simulink model "PersonFollower_TestModule"  (R2023b)
settings: Solver=FixedStepAuto  StartTime=0.0  StopTime=inf  FixedStep=1  RelTol=1e-3
model workspace (MAT data in the model file):
  SL_ROS_VariableLengthArrays_MaxSizes.CommonInfo.ArrayTruncateAction = 'EmitWarning'
  SL_ROS_VariableLengthArrays_MaxSizes.MsgTypeMap = containers.Map
  SL_ROS_VariableLengthArrays_MaxSizes.MsgTypeMap.serialization.keys = {'sensor_msgs/CompressedImage', 'sensor_msgs/LaserScan'}
  SL_ROS_VariableLengthArrays_MaxSizes.MsgTypeMap.serialization.values{1}(1).PropertyName = 'data'
  SL_ROS_VariableLengthArrays_MaxSizes.MsgTypeMap.serialization.values{1}(1).DataType = 'uint8'
  SL_ROS_VariableLengthArrays_MaxSizes.MsgTypeMap.serialization.values{1}(1).MaxLength = 300000
  SL_ROS_VariableLengthArrays_MaxSizes.MsgTypeMap.serialization.values{1}(2).PropertyName = 'format'
  SL_ROS_VariableLengthArrays_MaxSizes.MsgTypeMap.serialization.values{1}(2).DataType = 'uint8'
  SL_ROS_VariableLengthArrays_MaxSizes.MsgTypeMap.serialization.values{1}(2).MaxLength = 128
  SL_ROS_VariableLengthArrays_MaxSizes.MsgTypeMap.serialization.values{2}(1).PropertyName = 'intensities'
  SL_ROS_VariableLengthArrays_MaxSizes.MsgTypeMap.serialization.values{2}(1).DataType = 'single'
  SL_ROS_VariableLengthArrays_MaxSizes.MsgTypeMap.serialization.values{2}(1).MaxLength = 2000
  SL_ROS_VariableLengthArrays_MaxSizes.MsgTypeMap.serialization.values{2}(2).PropertyName = 'ranges'
  SL_ROS_VariableLengthArrays_MaxSizes.MsgTypeMap.serialization.values{2}(2).DataType = 'single'
  SL_ROS_VariableLengthArrays_MaxSizes.MsgTypeMap.serialization.values{2}(2).MaxLength = 2000
  SL_ROS_VariableLengthArrays_MaxSizes.MsgTypeMap.serialization.uniformity = 0
  SL_ROS_VariableLengthArrays_MaxSizes.MsgTypeMap.serialization.keyType = 'char'
  SL_ROS_VariableLengthArrays_MaxSizes.MsgTypeMap.serialization.valueType = 'any'
undefined symbols (not defined in the file or in its folder): angular, linear
libraries: ros2lib x6, simulink_extras x1, simulink x1
settings Model: Creator=bowen  LastModifiedBy=bowen
settings OptimizationCC: EnhancedBackFolding=on  PassReuseOutputArgsAs=Individual arguments  ZeroExternalMemoryAtStartup=off  ZeroInternalMemoryAtStartup=off  MaxStackSize=64  OptimizeBlockOrder=speed  DifferentSizesBufferReuse=on  OptimizationCustomize=off  EfficientTunableParamExpr=on
settings DebuggingCC: ParameterTunabilityLossMsg=error
settings SFSimCC: MATLABDynamicMemAlloc=off
settings RTWCC: Description=Embedded Coder  SystemTargetFile=ert.tlc  HardwareBoard=Robot Operating System 2 (ROS 2)  TLCOptions="-aInlineSetEventsForThisBaseRateFcn=TLC_FALSE -aSuppressMultiTaskScheduler=TLC_FALSE  -aRateBasedStepFcn=0"  TemplateMakefile=ert_default_tmf  Toolchain=Colcon Tools  TargetLang=C++
settings CodeAppCC: ForceParamTrailComments=on  IgnoreCustomStorageClasses=off  OperatorAnnotations=on  SimulinkDataObjDesc=on  SFDataObjDesc=on  InsertBlockDesc=on
settings ERTTargetCC: CodeInterfacePackaging=C++ class  RootIOFormat=Structure reference

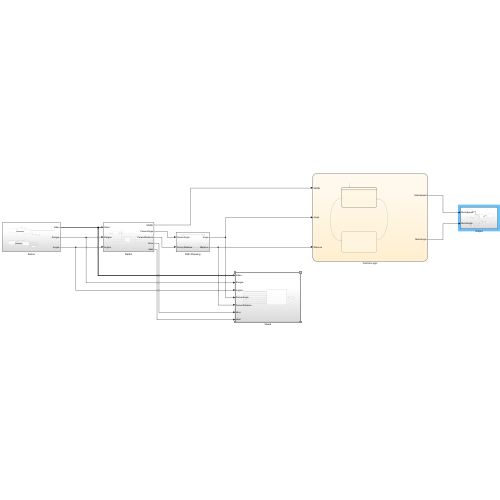
[thumbnail: Simulink's stored preview of the top-level diagram]
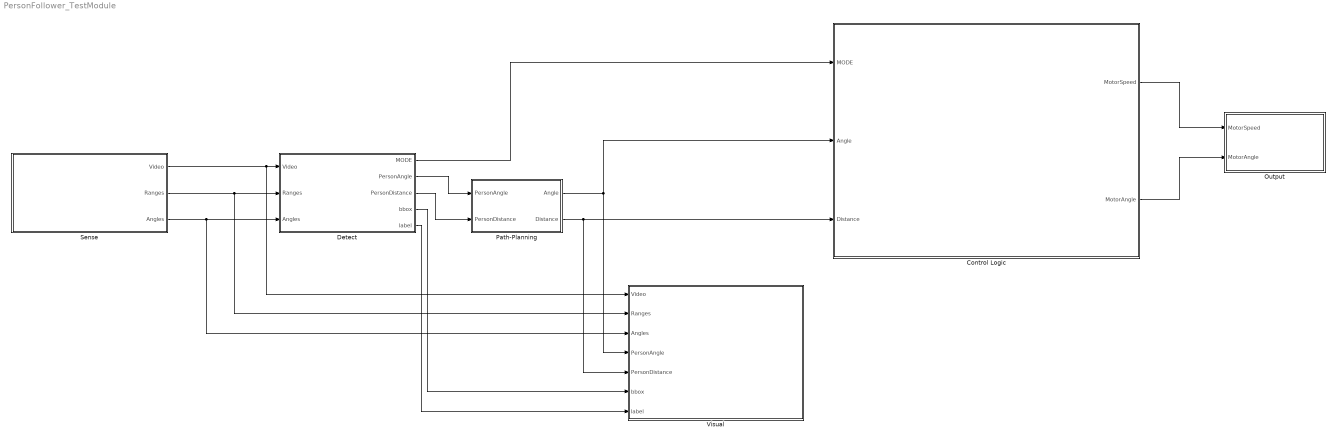
== system PersonFollower_TestModule ==
  Control Logic : Stateflow chart  TreatAsAtomicUnit=on
  Detect : Subsystem
  Output : Subsystem
  Path-Planning : Subsystem
  Sense : Subsystem
  Visual : Subsystem
  wires:
  Sense/1(Video) -> Visual/1(Video), Detect/1(Video)
  Sense/2(Ranges) -> Visual/2(Ranges), Detect/2(Ranges)
  Sense/3(Angles) -> Visual/3(Angles), Detect/3(Angles)
  Detect/1(MODE) -> Control Logic/1(MODE)
  Control Logic/1(MotorSpeed) -> Output/1(MotorSpeed)
  Control Logic/2(MotorAngle) -> Output/2(MotorAngle)
  Detect/2(PersonAngle) -> Path-Planning/1("PersonAngle ")
  Detect/3(PersonDistance) -> Path-Planning/2(PersonDistance)
  Path-Planning/1(Angle) -> Control Logic/2(Angle), Visual/4(PersonAngle)
  Path-Planning/2(Distance) -> Visual/5(PersonDistance), Control Logic/3(Distance)
  Detect/4(bbox) -> Visual/6(bbox)
  Detect/5(label) -> Visual/7(label)

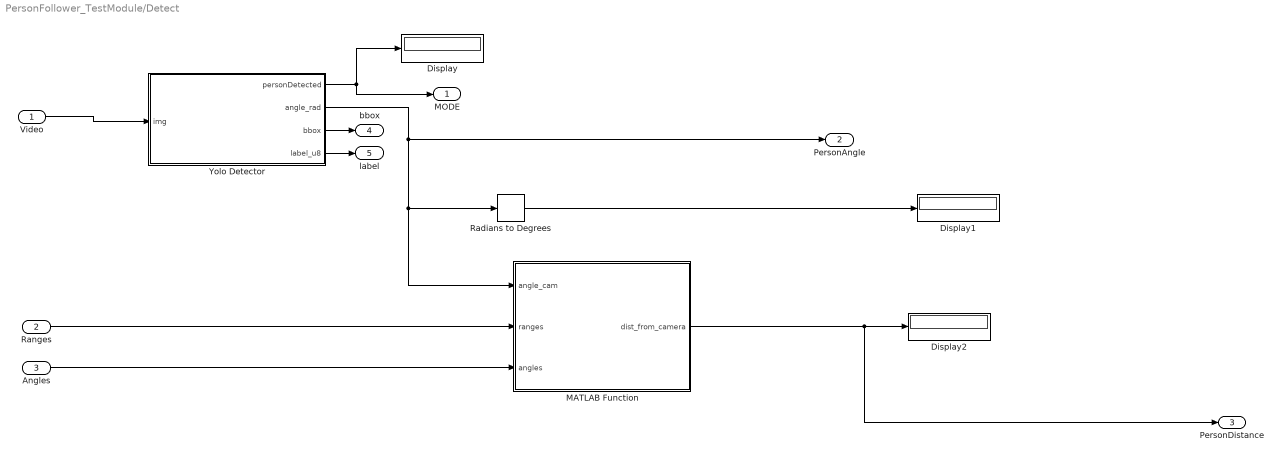
== system PersonFollower_TestModule/Detect ==
  Video : Inport
  Ranges : Inport  Port=2
  Angles : Inport  Port=3
  Display : Display
  Display1 : Display
  Display2 : Display
  MATLAB Function : MATLAB Function  TreatAsAtomicUnit=on
  Radians to Degrees : simulink_extras/Transformations/Radians to Degrees
  Yolo Detector : MATLAB Function  TreatAsAtomicUnit=on
  MODE : Outport
  PersonAngle : Outport  Port=2
  PersonDistance : Outport  Port=3
  bbox : Outport  Port=4
  label : Outport  Port=5
  wires:
  Video/1 -> Yolo Detector/1(img)
  Yolo Detector/1(personDetected) -> MODE/1, Display/1
  Yolo Detector/2(angle_rad) -> MATLAB Function/1(angle_cam), Radians to Degrees/1, PersonAngle/1
  Ranges/1 -> MATLAB Function/2(ranges)
  Angles/1 -> MATLAB Function/3(angles)
  Radians to Degrees/1 -> Display1/1
  MATLAB Function/1(dist_from_camera) -> PersonDistance/1, Display2/1
  Yolo Detector/3(bbox) -> bbox/1
  Yolo Detector/4(label_u8) -> label/1

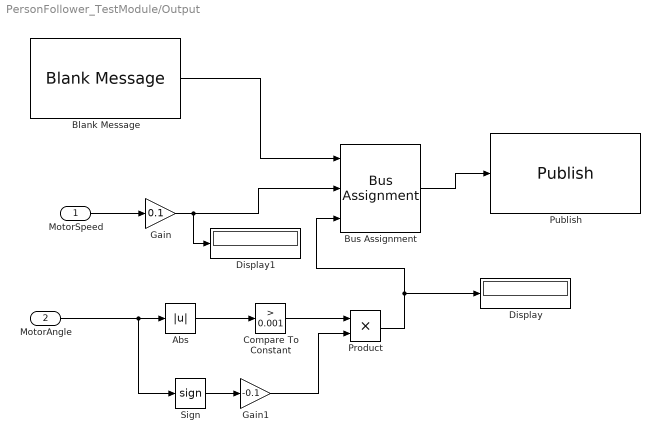
== system PersonFollower_TestModule/Output ==
  MotorSpeed : Inport
  MotorAngle : Inport  Port=2
  Abs : Abs  SaturateOnIntegerOverflow=off
  Blank Message : ros2lib/Blank Message  messageClass=Message  entityType=geometry_msgs/Twist  messageType=geometry_msgs/Twist  SampleTime=1
  Bus Assignment : BusAssignment  AssignedSignals=linear.x,angular.z
  Compare To Constant : simulink/Logic and Bit Operations/Compare To Constant  relop=>  const=0.001  OutDataTypeStr=boolean
  Display : Display
  Display1 : Display
  Gain : Gain  Gain=0.1
  Gain1 : Gain  Gain=-0.1
  Product : Product
  Publish : ros2lib/Publish  topicSource=Select from ROS network  topic=/controller/cmd_vel  messageType=geometry_msgs/Twist  QOSHistory=Keep last  QOSDepth=1  QOSReliability=Reliable  QOSDurability=Volatile
  Sign : Signum
  wires:
  Blank Message/1 -> Bus Assignment/1
  Bus Assignment/1 -> Publish/1
  Gain/1 -> Bus Assignment/2, Display1/1
  MotorSpeed/1 -> Gain/1
  MotorAngle/1 -> Sign/1, Abs/1
  Abs/1 -> Compare To Constant/1
  Sign/1 -> Gain1/1
  Compare To Constant/1 -> Product/1
  Gain1/1 -> Product/2
  Product/1 -> Display/1, Bus Assignment/3

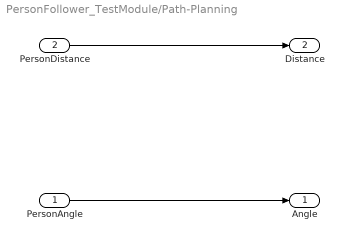
== system PersonFollower_TestModule/Path-Planning ==
  "PersonAngle " : Inport
  PersonDistance : Inport  Port=2
  Angle : Outport
  Distance : Outport  Port=2
  wires:
  PersonDistance/1 -> Distance/1
  "PersonAngle "/1 -> Angle/1

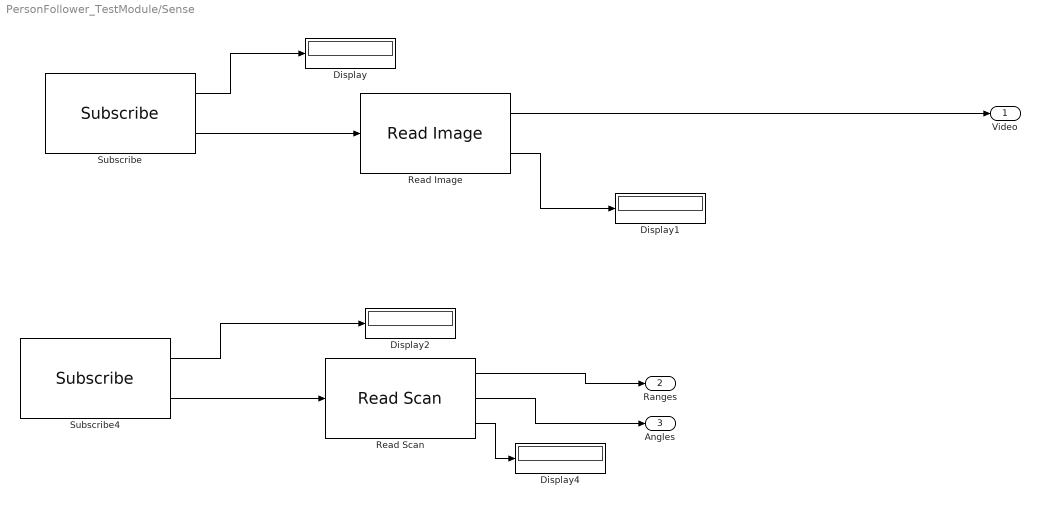
== system PersonFollower_TestModule/Sense ==
  Display{,1..2,4} (4 alike) : Display
  Read Image : ros2lib/Read Image  MaximumImageSize=[480, 640]  ImageEncoding=rgb8  ShowAlphaOutput=off  ShowErrorCodeOutput=on  VariableSizeOutputs=on
  Read Scan : ros2lib/Read Scan  MaximumArrayLength=1080  ShowAnglesOutput=on  ShowIntensityOutput=off  ShowErrorCodeOutput=on  VariableSizeOutputs=off
  Subscribe : ros2lib/Subscribe  topicSource=Select from ROS network  topic=/depth_cam/rgb/image_raw/compressed  messageType=sensor_msgs/CompressedImage  sampleTime=-1  QOSHistory=Keep last  QOSDepth=1  QOSReliability=Best effort  QOSDurability=Volatile
  Subscribe4 : ros2lib/Subscribe  topicSource=Select from ROS network  topic=/scan  messageType=sensor_msgs/LaserScan  sampleTime=-1  QOSHistory=Keep last  QOSDepth=1  QOSReliability=Best effort  QOSDurability=Volatile
  Video : Outport
  Ranges : Outport  Port=2
  Angles : Outport  Port=3
  wires:
  Read Image/2 -> Display1/1
  Subscribe/2 -> Read Image/1
  Subscribe/1 -> Display/1
  Read Image/1 -> Video/1
  Subscribe4/2 -> Read Scan/1
  Read Scan/3 -> Display4/1
  Read Scan/1 -> Ranges/1
  Read Scan/2 -> Angles/1
  Subscribe4/1 -> Display2/1

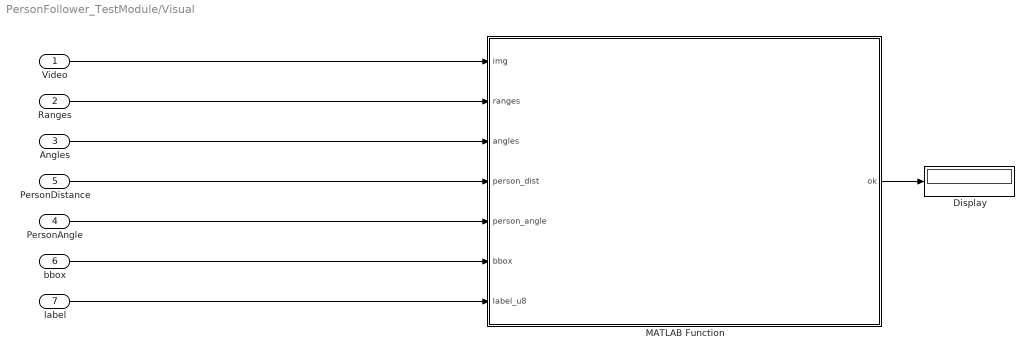
== system PersonFollower_TestModule/Visual ==
  Video : Inport
  Ranges : Inport  Port=2
  Angles : Inport  Port=3
  PersonAngle : Inport  Port=4
  PersonDistance : Inport  Port=5
  bbox : Inport  Port=6
  label : Inport  Port=7
  Display : Display
  MATLAB Function : MATLAB Function  TreatAsAtomicUnit=on
  wires:
  Video/1 -> MATLAB Function/1(img)
  Ranges/1 -> MATLAB Function/2(ranges)
  Angles/1 -> MATLAB Function/3(angles)
  PersonAngle/1 -> MATLAB Function/5(person_angle)
  PersonDistance/1 -> MATLAB Function/4(person_dist)
  MATLAB Function/1(ok) -> Display/1
  bbox/1 -> MATLAB Function/6(bbox)
  label/1 -> MATLAB Function/7(label_u8)

== matlab function PersonFollower_TestModule/Detect/MATLAB Function ==
  data: angle_cam input; dist_from_camera output; ranges input; angles input
function dist_from_camera = lidar_distance_on_bearing(angle_cam, ranges, angles)
%#codegen
% Estimate camera->target distance along a YOLO-provided bearing using LiDAR data.
% Inputs:
%   angle_cam : radians (bearing from YOLO)
%   ranges(:) : LiDAR range readings (m)
%   angles(:) : beam angles corresponding to 'ranges' (radians)
% Output:
%   dist_from_camera : fused distance from camera to target (m), NaN if none.

% === Local parameters (tune as needed) ===
cam_y_offset_m = -0.07;    % camera is 7 cm behind LiDAR (forward-negative)
yaw_offset     = 0.0;      % calibration offset between camera and LiDAR (rad)
threshold_m    = 0.05;     % lateral band threshold (m) for intersection
range_min      = 0.05;     % min valid range (m)

% --- Basic checks ---
dist_from_camera = NaN;
if isempty(ranges) || isempty(angles)
    return;
end

% --- Filter valid points ---
mask = isfinite(ranges) & (ranges > range_min);
if ~any(mask)
    return;
end
r = double(ranges(mask));
th = double(angles(mask));

% --- Convert polar → plot frame (same as SensorFusion.m) ---
x_plot = r .* sin(th);    % right
y_plot = -r .* cos(th);   % forward

% --- Camera → LiDAR bearing ---
thetaLid = angle_cam - yaw_offset;

% --- Find intersection distance from LiDAR ---
r_from_lidar = localFindRayIntersection(x_plot, y_plot, thetaLid, threshold_m);

% --- Convert LiDAR→target → camera→target distance ---
if ~isnan(r_from_lidar)
    angle_at_lidar = pi/2 - thetaLid; % consistent with plotting frame
    dist_sq = r_from_lidar^2 + cam_y_offset_m^2 - ...
              2 * r_from_lidar * abs(cam_y_offset_m) * cos(angle_at_lidar);
    if dist_sq >= 0
        dist_from_camera = sqrt(dist_sq);
    end
end
end


% ==== Local helper ====
function range_at_intersection = localFindRayIntersection(x, y, target_angle, threshold_m)
% Robustly estimate distance along the ray defined by 'target_angle'

range_at_intersection = NaN;
if isempty(x)
    return;
end

dx = -sin(target_angle);
dy =  cos(target_angle);

% Lateral distance band and forward filter
perp  = abs(dx.*y - dy.*x);
ahead = (dx.*x + dy.*y) > 0;
cand  = (perp <= threshold_m) & ahead;
if ~any(cand)
    return;
end

rc = hypot(x(cand), y(cand));
rc = rc(isfinite(rc) & rc > 0);
if isempty(rc)
    return;
end

% Robust filtering
rmed = median(rc);
madv = median(abs(rc - rmed));
if madv > 0
    inlier = abs(rc - rmed) <= 3 * 1.4826 * madv;
    rc = rc(inlier);
end

if numel(rc) >= 5
    rc = sort(rc);
    n = numel(rc);
    lo = ceil(0.10*n);
    hi = floor(0.90*n);
    if lo < 1, lo = 1; end
    if hi > n, hi = n; end
    rc = rc(lo:hi);
    range_at_intersection = mean(rc);
else
    range_at_intersection = min(rc);
end
end

== matlab function PersonFollower_TestModule/Detect/Yolo Detector ==
  data: img input; personDetected output; angle_rad output; bbox output; label_u8 output
function [personDetected, angle_rad, bbox, label_u8] = yolo_person_bearing_block(img)
%#codegen
% Outputs:
%   personDetected : uint8  (1 if person found, else 0)
%   angle_rad      : double (thetaCam in radians; NaN if none)
%   bbox           : 1x4 double [x y w h] (zeros if none)
%   label_u8       : 1x32 uint8 ASCII bytes (padded with spaces=32)

coder.extrinsic('yolo_person_bearing_wrapper');

% ---- Fixed-size, fixed-type pre-inits (lets Simulink infer ports) ----
personDetected = uint8(0);
angle_rad      = NaN;
bbox           = zeros(1,4);                % double [1x4]
label_u8       = uint8(32*ones(1,32));      % uint8 [1x32], spaces

% Direct assign from the extrinsic wrapper
[personDetected, angle_rad, bbox, label_u8] = yolo_person_bearing_wrapper(img);
end

== stateflow chart PersonFollower_TestModule/Control Logic ==
  state Idle1
    entry:
    MotorSpeed = 0
    MotorAngle = 0
  state Follow
    entry:
    MotorSpeed = 1
    MotorAngle = Angle
  (default) -> Idle1
  Idle1 -> Follow : [MODE==1 && Distance > 0.75]
  Follow -> Idle1 : [MODE==0 || Distance < 0.75]
  data: MODE input; Angle input; MotorSpeed output; MotorAngle output; Distance input

== matlab function PersonFollower_TestModule/Visual/MATLAB Function ==
  data: img input; ranges input; angles input; person_dist input; person_angle input; ok output; bbox input; label_u8 input
function ok = visualizer_popup(img, ranges, angles, person_dist, person_angle, bbox, label_u8)
%#codegen
% One popup: video (left) + 3D LiDAR scene (right) with distance overlay.
% Bounding box inputs are ignored.
%
% Inputs:
%   img            : HxWx3 uint8 RGB
%   ranges(:)      : double LiDAR ranges (m)
%   angles(:)      : double LiDAR angles (rad)
%   person_dist    : double camera->target distance (m), NaN if none
%   person_angle   : double bearing (rad)
%   bbox(1x4)      : (IGNORED) double [x y w h]
%   label_u8(1x32) : (IGNORED) uint8 ASCII text
% Output:
%   ok             : uint8 (always 1)

% Extrinsic graphics & annotation functions (simulation only)
coder.extrinsic('figure','subplot','imshow','ishghandle','cla','hold','grid');
coder.extrinsic('scatter3','patch','title','xlabel','ylabel','zlabel');
coder.extrinsic('xlim','ylim','zlim','axis','view','set','get','image','insertShape','insertText');

ok = uint8(1);

% ---- Persistent graphics handles (never assign []) ----
persistent fig axImg ax3D hImg hLidarScan hPerson hRay hCar

% Create figure & primitives the first time
if isempty(fig)
    fig = figure('Name','Sensor Fusion 3D Visualizer','NumberTitle','off', ...
                 'Position',[100,100,1280,600]);
    % Left: camera pane
    axImg = subplot(1,2,1,'Parent',fig);
    imshow(uint8(zeros(480,640,3)),'Parent',axImg);
    hImg = image(axImg,'CData',img);
    title(axImg,'Camera');
    
    % Right: 3D pane
    ax3D = subplot(1,2,2,'Parent',fig);
    cla(ax3D); hold(ax3D,'on'); grid(ax3D,'on');
    title(ax3D,'LiDAR 3D View (Drag to rotate)');
    xlabel(ax3D,'X right (m)'); ylabel(ax3D,'Y fwd (m)'); zlabel(ax3D,'Z (m)');
    
    % --- Car Body (unchanged) ---
    cw = 0.2; cl = 0.3; ch = 0.3;
    hx = cw/2; hy = cl/2; hz = ch;
    V_car = [ -hx, -hy, 0;  +hx, -hy, 0;  +hx, +hy, 0;  -hx, +hy, 0; ...
              -hx, -hy, hz; +hx, -hy, hz; +hx, +hy, hz; -hx, +hy, hz ];
    F_car = [ 1 2 3 4; 5 6 7 8; 1 2 6 5; 2 3 7 6; 3 4 8 7; 4 1 5 8 ];
    hCar = patch(ax3D, 'Faces',F_car, 'Vertices',V_car, ...
                 'FaceColor',[0 0.4 1], 'FaceAlpha',0.8, 'EdgeColor','k');

    % --- Primitives (unchanged) ---
    hLidarScan = scatter3(ax3D, NaN,NaN,NaN, 10, 'b', 'filled');
    
    % --- MODIFIED: Define Faces ONCE during initialization ---
    F_person = [ 1 2 3 4; 5 6 7 8; 1 2 6 5; 2 3 7 6; 3 4 8 7; 4 1 5 8 ];
    hPerson   = patch(ax3D, 'Faces',F_person, 'Vertices',NaN(8,3), ...
                      'FaceColor',[1 0 0], 'FaceAlpha',0.35, 'EdgeColor','none', ...
                      'Visible','off');
    
    F_ray = [1 2 3 4];
    hRay      = patch(ax3D, 'Faces',F_ray, 'Vertices',NaN(4,3), ...
                      'FaceColor',[1 1 0], 'FaceAlpha',0.35, 'EdgeColor','none', ...
                      'Visible','off');
    
    % --- Set Standard Isometric View (unchanged) ---
    view(ax3D,[-35 25]); % Standard 3D view
    
    % --- Set initial limits (unchanged) ---
    xlim(ax3D,[-5 5]); ylim(ax3D,[-0.5 5]); zlim(ax3D,[0 3]);
    
else
    % If user closed the window, skip this tick (Simulink will recreate)
    if ~ishghandle(fig)
        return;
    end
end

% ---------- LEFT: video with overlay ----------
% (This section is unchanged)
img_to_show = img;
haveDist = isfinite(person_dist) && (person_dist > 0) && isfinite(person_angle);
if coder.target('MATLAB')
    overlay_drawn_dist = false;
    x_pos = 20;
    y_pos = 30;
    if haveDist
        overlay_drawn_dist = true;
        ang_deg = person_angle*(180/pi);
        txt = sprintf('dist: %.2f m @ %.1f deg', person_dist, ang_deg);
        img_to_show = insertText(img_to_show,[x_pos, y_pos],txt, ...
            'FontSize',18,'BoxOpacity',0.6,'TextColor','black','BoxColor','yellow');
    end
    if ~overlay_drawn_dist
        img_to_show = insertText(img_to_show, [x_pos, y_pos], 'No Target Detected', ...
            'FontSize', 18, 'BoxOpacity', 0.6, 'TextColor', 'white', 'BoxColor', 'red');
    end
end
set(hImg,'CData',img_to_show);

% ---------- RIGHT: 3D scene ----------
if ~isempty(ranges) && ~isempty(angles)
    ranges = double(ranges(:));
    angles = double(angles(:));
    mask = isfinite(ranges) & (ranges > 0.05);
    if any(mask)
        r  = ranges(mask);
        th = angles(mask);
        
        x = r .* sin(th);     % right
        y = -r .* cos(th);    % forward
        
        set(hLidarScan,'XData',x,'YData',y,'ZData',ones(size(x))*0.01,'Visible','on');

        % person box + ground strip if we have a target
        if haveDist
            px = person_dist * sin(person_angle);
            py = person_dist * cos(person_angle);
            
            % --- MODIFIED: Set person height to 1.5m ---
            bw = 0.4; bh = 0.4; hz = 1.5;  hx = bw/2; hy = bh/2; 
            
            V = [ px-hx, py-hy, 0;
                  px+hx, py-hy, 0;
                  px+hx, py+hy, 0;
                  px-hx, py+hy, 0;
                  px-hx, py-hy, hz;
                  px+hx, py-hy, hz;
                  px+hx, py+hy, hz;
                  px-hx, py+hy, hz ];
            
            % --- MODIFIED (FAST): Only update Vertices, not Faces ---
            set(hPerson,'Vertices',V,'Visible','on');
            
            % ground strip (“ray”)
            w = 0.5;  L = min(person_dist,5);
            dxr =  sin(person_angle);  dyr =  cos(person_angle);
            pxn = -dyr;                pyn =  dxr;
            A = [0 + (w/2)*pxn, 0 + (w/2)*pyn, 0.01];
            B = [0 - (w/2)*pxn, 0 - (w/2)*pyn, 0.01];
            C = [L*dxr - (w/2)*pxn, L*dyr - (w/2)*pyn, 0.01];
            D = [L*dxr + (w/2)*pxn, L*dyr + (w/2)*pyn, 0.01];
            
            % --- MODIFIED (FAST): Only update Vertices, not Faces ---
            set(hRay,'Vertices',[A;B;C;D],'Visible','on');
        else
            set(hPerson,'Visible','off'); 
            set(hRay,'Visible','off');
        end
        
        xlim(ax3D,[-5 5]); ylim(ax3D,[-0.5 5]); zlim(ax3D,[0 3]);
        
    else
        set(hLidarScan,'Visible','off');
        set(hPerson,'Visible','off'); set(hRay,'Visible','off');
    end
end
end
